simulink model "sf_fromworkspace"  (Simulink 6.0)
settings: Solver=ode45  StartTime=0.0  StopTime=100  MaxStep=.1  RelTol=1e-3
PreLoadFcn:
  | eval('load r12mlworkspace')
values from neighbouring files (symbols this model uses):
  delay = 20    [r12mlworkspace.mat]
  gain = 5    [r12mlworkspace.mat]
CloseFcn:
  | evalin('base','clear delay gain;')
settings Model: CovMetricSettings=dcmtr  Creator=The MathWorks Inc.  LastModifiedBy=batserve  ExtModeAutoUpdateStatusClock=off
settings DataIOCC: SaveTime=off  SignalLoggingName=sigsOut
settings OptimizationCC: BooleanDataType=off
settings DebuggingCC: CheckExecutionContextPreStartOutputMsg=on  CheckExecutionContextRuntimeOutputMsg=on  SolverPrmCheckMsg=none
settings HardwareCC: TargetUnknown=on

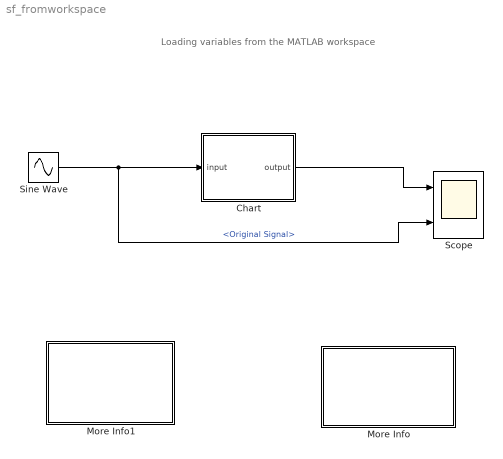
== system sf_fromworkspace ==
  note: Loading variables from the MATLAB workspace
  Chart : Stateflow chart  TreatAsAtomicUnit=on  PropExecContextAcrossSSBoundary=on
  More Info : Subsystem  PropExecContextAcrossSSBoundary=on
      mask Display: disp('Double click\nhere for\ninformation on\nthis demonstration')
  More Info1 : Subsystem  PropExecContextAcrossSSBoundary=on
      settings: OpenFcn=simcad(bdroot);
      mask Display: disp('Double click\nhere for\nSimulink\Stateflow\n Help')
  Scope : Scope  NumInputPorts=2
      settings: TimeRange=100  YMin=-5~-1  YMax=5~1
  Sine Wave : Sin  SampleTime=0
  wires:
  Sine Wave/1 -> Chart/1(input), Scope/2  "<Original Signal>"
  Chart/1(output) -> Scope/1

== system sf_fromworkspace/More Info ==
  note: Loading MATLAB variables
  note: The purpose of this demonstration is to illustrate how variables in your Stateflow chart can be
      | defined and initialized from the MATLAB workspace. You are also able to select
      | the 'Initialize From Workspace' property of the local variable.
      |
      | In this particular example, we initialize two variables from the MATLAB workspace: 'gain' and 'delay'.
      | The variables are initialized from the workspace by setting the 'Initialize From'  property.
      |
      | The 'gain' variable is used to determine the amplitude of the input sine wave and the 'delay' variable
      | is used to suppress the output of the sine wave for a certain amount of time.
      |
      | In this particular model, a graphical user interface (GUI) was also created using GUIDE to allow easy
      | access to the variabls that are definied in the workspace. This is not necessary since the variables can
      | simply be changed directly from the workspace. For example, changing the gain value to '9' using the GUI is
      | equivalent to running the following command at the MATLAB command line:
      |
      | >> gain = 9;

== system sf_fromworkspace/More Info1 ==

== stateflow chart Chart ==
  state A
    output=0;
  state B
    du: output=gain*input;
  note: The following variables are initialized
      | from the MATLAB workspace:
      |
      | gain    =  5
      | delay   =  20 (in seconds)
  A -> B : [t>delay]
  (default) -> A
  data: gain local double; input input double; output output double; delay local double
